simulink model "HouseThermalDataProducerKafka"  (R2019b)
settings: Solver=FixedStepAuto  StartTime=0.0  StopTime=24*60*60  FixedStep=.1  MaxStep=50  RelTol=1e-3  AbsTol=1e-3
PreLoadFcn:
  | %Load Input Data
  | prepareInputData
  | 
  | % Time step and initial conditions
  | PIDFault = false;
  | BlockageOn = false;
  | Ts = 5;
  | load InitialConditions.mat
  | 
  | % Walls
  | lenHouse   = 30;          % House length [m]
  | widHouse   = 10;          % House width [m]
  | htHouse     = 4;            % House height [m]
  | LWall           = 0.2;         % Wall thickness [m]
  | wallDensity = 1920;      % Density [kg/m^3]
  | c_wall          = 835;        % Specific heat [J/kg/K]
  | kWall            = 0.038;    % Thermal conductivity [W/m/K]
  | 
  | % Windows
  | n1_window       = 3;          % Number or windows in room 1
  | n2_window       = 2;          % Number or windows in room 2
  | n3_window       = 2;          % Number or windows in room 3
  | n4_window       = 2;          % Number or windows in room 4
  | htWindows       = 1;          % Height of windows [m]
  | widWindows      = 1;          % Width of windows  [m]
  | LWindow           = 0.01;     % Thickenss of windows [m]
  | windowDensity = 2700;    % Density [kg/m^3]
  | c_window          = 840;      % Specific heat [J/kg/K]
  | kWindow           = 0.78;     % Thermal conductivity [W/m/K]
  | 
  | 
  | % Roof
  | pitRoof         = 40/180/pi;   % Roof pitch (40 deg)
  | LRoof           = 0.2;             % Roof thickness [m]
  | roofDensity = 32;              % Roof density (Glass fiber) [kg/m^3]
  | c_roof          = 835;            % Specific heat [J/kg/K]
  | kRoof           = 0.038;         % Thermal conductivity [W/m/K]
  | 
  | % Radiators
  | %% Exchange area with air
  | S_radiator1 = 5;     % [m^2]
  | S_radiator2 = 5;     % [m^2]
  | S_radiator3 = 5;     % [m^2]
  | S_radiator4 = 5;     % [m^2]
  | %% Convective heat transfer coefficient radiator -> room
  | h_radiator1 = 100;  %  [W/(m^2 * K)]
  | h_radiator2 = 100;  %  [W/(m^2 * K)]
  | h_radiator3 = 100;  %  [W/(m^2 * K)]
  | h_radiator4 = 100;  %  [W/(m^2 * K)]
  | 
  | % Convective heat transfer coefficients [W/M^2/K]
  | h_air_wall         = 18;    % Indoor air->walls
  | h_wall_atm       = 20;   % Walls -> atmosphere
  | h_air_window    = 16;   % Indoor air -> windows
  | h_window_atm = 18;    % Windows -> atmosphere
  | h_air_roof         = 8;   % Indoor air -> roof
  | h_roof_atm      = 20;    % Roof -> atmosphere
  | 
  | %Air
  | c_air = 1005.4;         % cp of air at 273 K [J/(kg*K]
  | 
  | % Leakage fraction
  | leak_roof_percent = 0.1;     % Leakage through roof
  | leak_wall_percent  = 0.15;  % Leakage through walls
  | leak_win_percent  = 0.2;     % Leakage through windows
  | 
  | % Roof
  | roofArea =  2* (widHouse/(2*cos(pitRoof))*lenHouse);
  | 
  | %Rooms
  | %% Room 1
  | area_window_room1 = 3 * 1 *1;
  | area_wall_room1 = (lenHouse*3/5 *htHouse+widHouse*2/3*htHouse) - area_window_room1;
  | area_roof_room1 = roofArea/4;
  | 
  | %% Room 2
  | area_window_room2 = 2 * 1 *1;
  | area_wall_room2 = (lenHouse*3/5*htHouse+widHouse/3*htHouse) - area_window_room2;
  | area_roof_room2 = roofArea/4;
  | 
  | %% Room 3
  | area_window_room3 =2* 1 *1;
  | area_wall_room3 = (lenHouse*2/5*htHouse+widHouse*2/3*htHouse) - area_window_room3;
  | area_roof_room3 = roofArea/4;
  | 
  | %% Room 4
  | area_window_room4 = 2 * 1 *1;
  | area_wall_room4 = (lenHouse*2/5*htHouse+widHouse/3*htHouse) - area_window_room4;
  | area_roof_room4 = roofArea/4;
  | 
  | % Cost estimation
  | % Assume the cost of natural gas is $8.50 per thousand cubic feet (Mcf): $8.50 per 1000 cf
  | % cost = $8.50/(1000 * 0.02831) m^3
  | cost = 8.50/(1000 * 0.02831);
  | % Natural gas density ~ 0.9 kg/m^3
  | NG_density = 0.9;
undefined symbols (not defined in the file or in its folder): localhost
libraries: HouseThermal_lib x3
Description:
  | House Heating System
  | 
  | Copyright 2008-2018 The MathWorks, Inc.
settings Model: FPTRunName=Active  ExtModeTrigMode=oneshot  ExtModeArmWhenConnect=off  ExtModeAutoUpdateStatusClock=off  Creator=MathWorks  LastModifiedBy=asolland
settings SolverCC: AutoScaleAbsTol=off  ZeroCrossControl=DisableAll
settings DataIOCC: ExternalInput=ForwardTTSim, AmbientTTSim, ReturnTTSim  InitialState=[]  MaxDataPoints=20000  LoadExternalInput=on  SaveFormat=Array  DSMLogging=off  ReturnWorkspaceOutputs=off
settings OptimizationCC: BlockReduction=off  BooleanDataType=off  DefaultParameterBehavior=Inlined  EnhancedBackFolding=on  PassReuseOutputArgsAs=Individual arguments  ExpressionDepthLimit=2147483647  InitFltsAndDblsToZero=on  BufferReusableBoundary=off  OptimizeBlockOrder=speed  DifferentSizesBufferReuse=on  OptimizationCustomize=off  EfficientTunableParamExpr=on
settings DebuggingCC: SaveWithParameterizedLinksMsg=none  UnderspecifiedInitializationDetection=Classic  MergeDetectMultiDrivingBlocksExec=none  SignalResolutionControl=TryResolveAllWithWarning  MultiTaskDSMMsg=warning  MultiTaskCondExecSysMsg=none  IntegerOverflowMsg=none  ParameterTunabilityLossMsg=error  BusObjectLabelMismatch=none  AllowSymbolicDim=off  StateNameClashWarn=warning  PregeneratedLibrarySubsystemCodeDiagnostic=none  SFUnexpectedBacktrackingDiag=warning  SFNoUnconditionalDefaultTransitionDiag=warning  SFExecutionAtInitializationDiag=none  IntegerSaturationMsg=none  ArithmeticOperatorsInVariantConditions=warning
settings HardwareCC: ProdBitPerPointer=32  ProdBitPerSizeT=32  ProdBitPerPtrDiffT=32  ProdLargestAtomicFloat=None  ProdIntDivRoundTo=Undefined  ProdEndianess=Unspecified  ProdWordSize=32  ProdHWDeviceType=32-bit Generic  TargetBitPerLong=64  TargetBitPerPointer=64  TargetBitPerSizeT=64  TargetBitPerPtrDiffT=64  TargetLongLongMode=on  TargetIntDivRoundTo=Zero  TargetEndianess=LittleEndian  TargetWordSize=64  TargetHWDeviceType=MATLAB Host  ProdEqTarget=off
settings ModelReferenceCC: PropagateSignalLabelsOutOfModel=off
settings SFSimCC: SimUseLocalCustomCode=off  SimParseCustomCode=off  MATLABDynamicMemAlloc=off  CustomCodeUndefinedFunction=UseInterfaceOnly
settings RTWCC: Description=Kafka Target  SystemTargetFile=kafkatarget.tlc  TemplateMakefile=ert_default_tmf  RTWUseLocalCustomCode=off  IncludeHyperlinkInReport=on
settings CodeAppCC: ForceParamTrailComments=on  IgnoreCustomStorageClasses=off  OperatorAnnotations=on  SimulinkDataObjDesc=on  SFDataObjDesc=on  InsertBlockDesc=on
settings STFCustomTargetCC: TargetLangStandard=C99 (ISO)  MultiwordLength=256  GenerateSampleERTMain=on  CombineOutputUpdateFcns=on  ERTCustomFileBanners=on  SupportContinuousTime=off  SupportNonInlinedSFcns=off  RemoveResetFunc=on  MATLABClassNameForMDSCustomization=Simulink.SoftwareTarget.ERTCustomization  UseToolchainInfoCompliant=on  SystemTargetFile=kafkatarget.tlc
settings ERTTargetCC: TargetLangStandard=C99 (ISO)  GenerateSampleERTMain=on  ParMdlRefBuildCompliant=off  CompOptLevelCompliant=off  ConcurrentExecutionCompliant=off  ModelStepFunctionPrototypeControlCompliant=off  CPPClassGenCompliant=off  InlinedParameterPlacement=NonHierarchical  ERTCustomFileTemplate=kafkatarget_process.tlc
settings ConfigComp: CovMetricSettings=dw  CovHtmlReporting=on  CovSaveCumulativeToWorkspaceVar=on  CovSaveSingleToWorkspaceVar=on  CovShowResultsExplorer=off  CovExternalEMLEnable=off  CovSFcnEnable=off
settings SimscapeCC: SimscapeLogDataHistory=20000  SimscapeUseOperatingPoints=on  SimscapeOperatingPoint=op

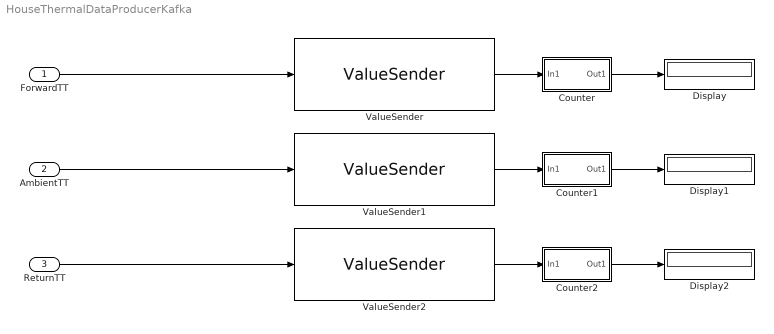
== system HouseThermalDataProducerKafka ==
  ForwardTT : Inport  Interpolate=off
  AmbientTT : Inport  Port=2  Interpolate=off
  ReturnTT : Inport  Port=3  Interpolate=off
  Counter : Subsystem
  Counter1 : Subsystem
  Counter2 : Subsystem
  Display : Display
  Display1 : Display
  Display2 : Display
  ValueSender : HouseThermal_lib/ValueSender  prmBroker=localhost:9092  prmTopicName=iot.forwardtemp.house  prmTopicKey=house1
  ValueSender1 : HouseThermal_lib/ValueSender  prmBroker=localhost:9092  prmTopicName=iot.ambienttemp.house  prmTopicKey=house1
  ValueSender2 : HouseThermal_lib/ValueSender  prmBroker=localhost:9092  prmTopicName=iot.returntemp.house  prmTopicKey=house1
  wires:
  AmbientTT/1 -> ValueSender1/1
  ReturnTT/1 -> ValueSender2/1
  ForwardTT/1 -> ValueSender/1
  ValueSender/1 -> Counter/1(In1)
  Counter/1(Out1) -> Display/1
  Counter1/1(Out1) -> Display1/1
  Counter2/1(Out1) -> Display2/1
  ValueSender1/1 -> Counter1/1(In1)
  ValueSender2/1 -> Counter2/1(In1)

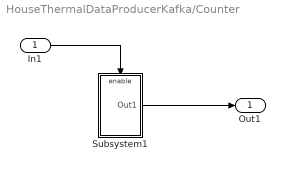
== system HouseThermalDataProducerKafka/Counter ==
  In1 : Inport
  Subsystem1 : Subsystem
  Out1 : Outport  VectorParamsAs1DForOutWhenUnconnected=off
  wires:
  Subsystem1/1(Out1) -> Out1/1
  In1/1 -> Subsystem1/Enable

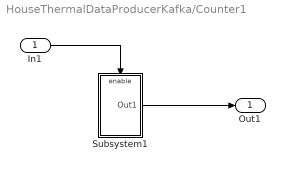
== system HouseThermalDataProducerKafka/Counter1 ==
  In1 : Inport
  Subsystem1 : Subsystem
  Out1 : Outport  VectorParamsAs1DForOutWhenUnconnected=off
  wires:
  In1/1 -> Subsystem1/Enable
  Subsystem1/1(Out1) -> Out1/1

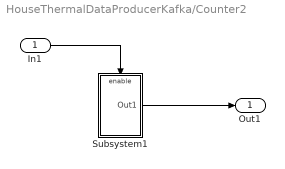
== system HouseThermalDataProducerKafka/Counter2 ==
  In1 : Inport
  Subsystem1 : Subsystem
  Out1 : Outport  VectorParamsAs1DForOutWhenUnconnected=off
  wires:
  Subsystem1/1(Out1) -> Out1/1
  In1/1 -> Subsystem1/Enable

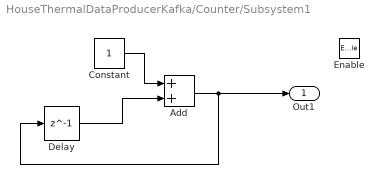
== system HouseThermalDataProducerKafka/Counter/Subsystem1 ==
  Enable : EnablePort
  Add : Sum
  Constant : Constant
  Delay : Delay  DelayLength=1
  Out1 : Outport  VectorParamsAs1DForOutWhenUnconnected=off
  wires:
  Constant/1 -> Add/1
  Delay/1 -> Add/2
  Add/1 -> Delay/1, Out1/1

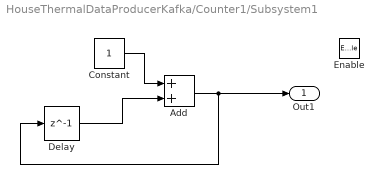
== system HouseThermalDataProducerKafka/Counter1/Subsystem1 ==
  Enable : EnablePort
  Add : Sum
  Constant : Constant
  Delay : Delay  DelayLength=1
  Out1 : Outport  VectorParamsAs1DForOutWhenUnconnected=off
  wires:
  Add/1 -> Out1/1, Delay/1
  Delay/1 -> Add/2
  Constant/1 -> Add/1

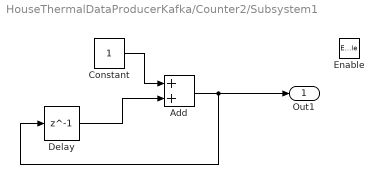
== system HouseThermalDataProducerKafka/Counter2/Subsystem1 ==
  Enable : EnablePort
  Add : Sum
  Constant : Constant
  Delay : Delay  DelayLength=1
  Out1 : Outport  VectorParamsAs1DForOutWhenUnconnected=off
  wires:
  Constant/1 -> Add/1
  Delay/1 -> Add/2
  Add/1 -> Delay/1, Out1/1
